simulink model "oba"  (Simulink 7.9)
settings: Solver=ode4  StartTime=0.0  StopTime=50.0  FixedStep=0.01  RelTol=1e-3
settings Model: Creator=student  LastModifiedBy=student

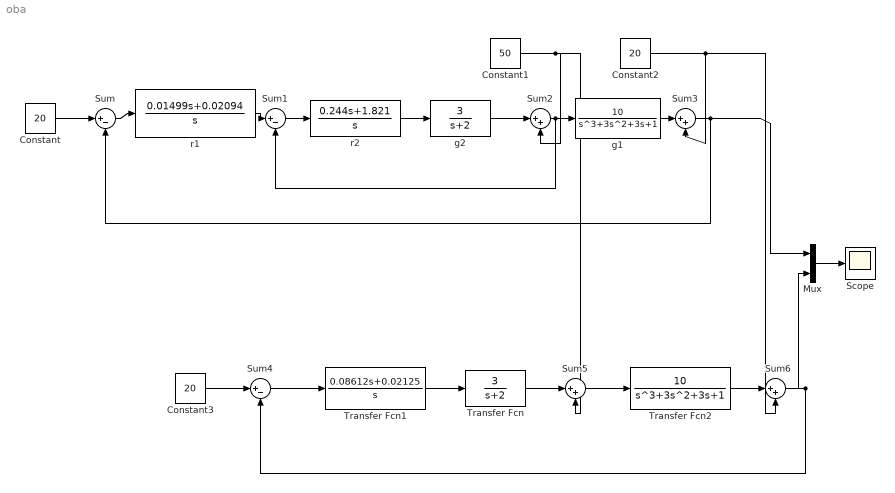
== system oba ==
  Constant : Constant  Value=20
  Constant1 : Constant  Value=50
  Constant2 : Constant  Value=20
  Constant3 : Constant  Value=20
  Mux : Mux  Inputs=2
  Scope : Scope
  Sum : Sum  Inputs=|+-
  Sum1 : Sum  Inputs=|+-
  Sum{2..3,5..6} (4 alike) : Sum  Inputs=|++
  Sum4 : Sum  Inputs=|+-
  Transfer Fcn : TransferFcn  Numerator=[3]  Denominator=[1 2]
  Transfer Fcn1 : TransferFcn  Numerator=[0.08612 0.02125]  Denominator=[1 0]
  Transfer Fcn2 : TransferFcn  Numerator=[10]  Denominator=[1 3 3 1]
  g1 : TransferFcn  Numerator=[10]  Denominator=[1 3 3 1]
  g2 : TransferFcn  Numerator=[3]  Denominator=[1 2]
  r1 : TransferFcn  Numerator=[0.01499 0.02094]  Denominator=[1 0]
  r2 : TransferFcn  Numerator=[0.244 1.821]  Denominator=[1 0]
  wires:
  Constant/1 -> Sum/1
  Sum/1 -> r1/1
  r1/1 -> Sum1/1
  Sum1/1 -> r2/1
  r2/1 -> g2/1
  g2/1 -> Sum2/1
  Constant1/1 -> Sum2/2, Sum5/2
  Sum2/1 -> g1/1, Sum1/2
  g1/1 -> Sum3/1
  Constant2/1 -> Sum3/2, Sum6/2
  Sum3/1 -> Sum/2, Mux/1
  Sum4/1 -> Transfer Fcn1/1
  Transfer Fcn1/1 -> Transfer Fcn/1
  Transfer Fcn2/1 -> Sum6/1
  Sum6/1 -> Sum4/2, Mux/2
  Transfer Fcn/1 -> Sum5/1
  Sum5/1 -> Transfer Fcn2/1
  Constant3/1 -> Sum4/1
  Mux/1 -> Scope/1
